simulink model "Ex2_enable"  (R2021a)
settings: Solver=FixedStepAuto  StartTime=0.0  StopTime=10.0  FixedStep=1e-3  MaxStep=1e-3  RelTol=1e-3
settings Model: Creator=reemb  LastModifiedBy=reemb

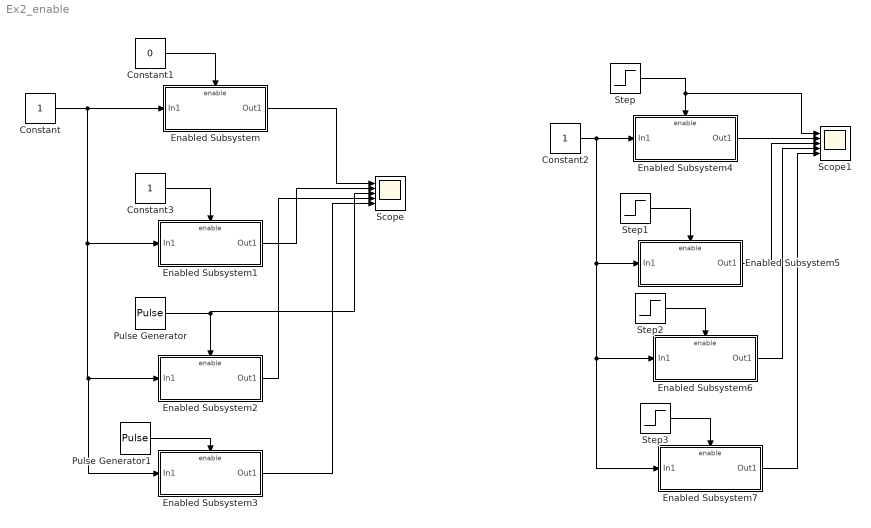
== system Ex2_enable ==
  Constant : Constant
  Constant1 : Constant  Value=0
  Constant2 : Constant
  Constant3 : Constant
  Enabled Subsystem : Subsystem  TreatAsAtomicUnit=on
  Enabled Subsystem1 : Subsystem  TreatAsAtomicUnit=on
  Enabled Subsystem2 : Subsystem  TreatAsAtomicUnit=on
  Enabled Subsystem3 : Subsystem  TreatAsAtomicUnit=on
  Enabled Subsystem4 : Subsystem  TreatAsAtomicUnit=on
  Enabled Subsystem5 : Subsystem  TreatAsAtomicUnit=on
  Enabled Subsystem6 : Subsystem  TreatAsAtomicUnit=on
  Enabled Subsystem7 : Subsystem  TreatAsAtomicUnit=on
  Pulse Generator : DiscretePulseGenerator  PulseType=Time based  PulseWidth=50
  Pulse Generator1 : DiscretePulseGenerator  PulseType=Time based  PulseWidth=50
  Scope : Scope  NumInputPorts=5
  Scope1 : Scope  NumInputPorts=5
  Step : Step  Before=-1  After=0  SampleTime=0
  Step1 : Step  Before=-1  SampleTime=0
  Step2 : Step  Before=1  After=2  SampleTime=0
  Step3 : Step  After=0.1  SampleTime=0
  wires:
  Constant1/1 -> Enabled Subsystem/Enable
  Enabled Subsystem/1(Out1) -> Scope/1
  Enabled Subsystem1/1(Out1) -> Scope/2
  Constant3/1 -> Enabled Subsystem1/Enable
  Constant/1 -> Enabled Subsystem/1(In1), Enabled Subsystem3/1(In1), Enabled Subsystem2/1(In1), Enabled Subsystem1/1(In1)
  Pulse Generator/1 -> Enabled Subsystem2/Enable, Scope/3
  Enabled Subsystem2/1(Out1) -> Scope/4
  Pulse Generator1/1 -> Enabled Subsystem3/Enable
  Enabled Subsystem3/1(Out1) -> Scope/5
  Step/1 -> Scope1/1, Enabled Subsystem4/Enable
  Enabled Subsystem4/1(Out1) -> Scope1/2
  Enabled Subsystem5/1(Out1) -> Scope1/3
  Step1/1 -> Enabled Subsystem5/Enable
  Step2/1 -> Enabled Subsystem6/Enable
  Enabled Subsystem6/1(Out1) -> Scope1/4
  Enabled Subsystem7/1(Out1) -> Scope1/5
  Step3/1 -> Enabled Subsystem7/Enable
  Constant2/1 -> Enabled Subsystem7/1(In1), Enabled Subsystem6/1(In1), Enabled Subsystem5/1(In1), Enabled Subsystem4/1(In1)

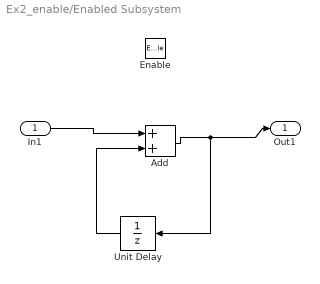
== system Ex2_enable/Enabled Subsystem ==
  In1 : Inport
  Enable : EnablePort
  Add : Sum
  Unit Delay : UnitDelay  SampleTime=-1  HasFrameUpgradeWarning=on
  Out1 : Outport
  wires:
  In1/1 -> Add/1
  Add/1 -> Unit Delay/1, Out1/1
  Unit Delay/1 -> Add/2

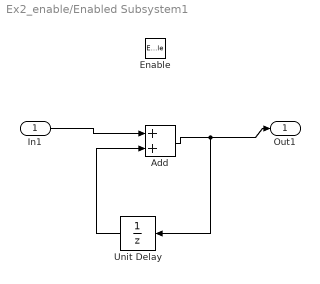
== system Ex2_enable/Enabled Subsystem1 ==
  In1 : Inport
  Enable : EnablePort
  Add : Sum
  Unit Delay : UnitDelay  SampleTime=-1  HasFrameUpgradeWarning=on
  Out1 : Outport
  wires:
  Unit Delay/1 -> Add/2
  Add/1 -> Out1/1, Unit Delay/1
  In1/1 -> Add/1

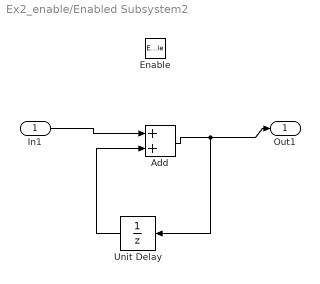
== system Ex2_enable/Enabled Subsystem2 ==
  In1 : Inport
  Enable : EnablePort
  Add : Sum
  Unit Delay : UnitDelay  SampleTime=-1  HasFrameUpgradeWarning=on
  Out1 : Outport
  wires:
  In1/1 -> Add/1
  Add/1 -> Unit Delay/1, Out1/1
  Unit Delay/1 -> Add/2

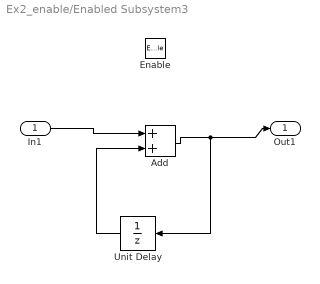
== system Ex2_enable/Enabled Subsystem3 ==
  In1 : Inport
  Enable : EnablePort  StatesWhenEnabling=reset
  Add : Sum
  Unit Delay : UnitDelay  SampleTime=-1  HasFrameUpgradeWarning=on
  Out1 : Outport
  wires:
  Unit Delay/1 -> Add/2
  Add/1 -> Out1/1, Unit Delay/1
  In1/1 -> Add/1

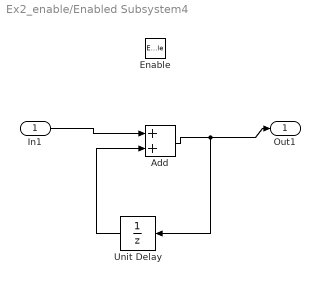
== system Ex2_enable/Enabled Subsystem4 ==
  In1 : Inport
  Enable : EnablePort
  Add : Sum
  Unit Delay : UnitDelay  SampleTime=-1  HasFrameUpgradeWarning=on
  Out1 : Outport
  wires:
  Unit Delay/1 -> Add/2
  Add/1 -> Out1/1, Unit Delay/1
  In1/1 -> Add/1

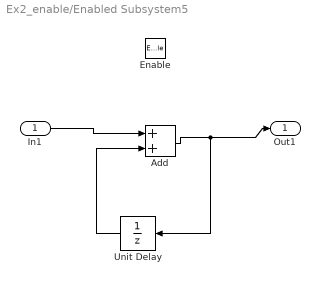
== system Ex2_enable/Enabled Subsystem5 ==
  In1 : Inport
  Enable : EnablePort
  Add : Sum
  Unit Delay : UnitDelay  SampleTime=-1  HasFrameUpgradeWarning=on
  Out1 : Outport
  wires:
  In1/1 -> Add/1
  Add/1 -> Unit Delay/1, Out1/1
  Unit Delay/1 -> Add/2

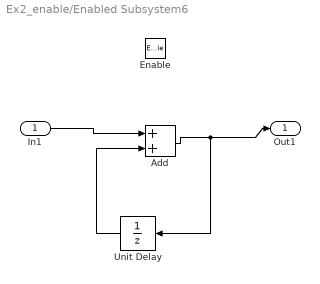
== system Ex2_enable/Enabled Subsystem6 ==
  In1 : Inport
  Enable : EnablePort
  Add : Sum
  Unit Delay : UnitDelay  SampleTime=-1  HasFrameUpgradeWarning=on
  Out1 : Outport
  wires:
  Unit Delay/1 -> Add/2
  Add/1 -> Out1/1, Unit Delay/1
  In1/1 -> Add/1

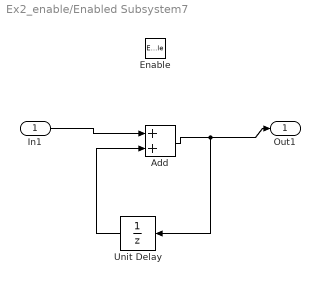
== system Ex2_enable/Enabled Subsystem7 ==
  In1 : Inport
  Enable : EnablePort
  Add : Sum
  Unit Delay : UnitDelay  SampleTime=-1  HasFrameUpgradeWarning=on
  Out1 : Outport
  wires:
  In1/1 -> Add/1
  Add/1 -> Unit Delay/1, Out1/1
  Unit Delay/1 -> Add/2
